simulink model "Problem11"  (R2020a)
settings: Solver=FixedStepDiscrete  StartTime=0.0  StopTime=10.0  FixedStep=1  RelTol=1e-3
settings Model: NumberOfSteps=10  Creator=shweta  LastModifiedBy=shweta

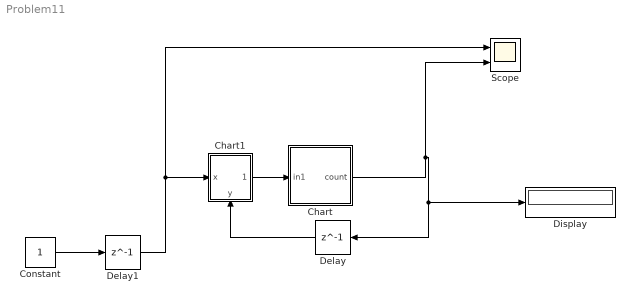
== system Problem11 ==
  Chart : Stateflow chart  TreatAsAtomicUnit=on
  Chart1 : Stateflow chart  TreatAsAtomicUnit=on
      settings: PortSchema="{\"entries\":[{\"content\":{\"sides\":[{\"content\":{\"connectorIds\":[\"In1\"]},\"type\":\"ConnectorPlacement.EquallySpacedRectSide\",\"uuid\":\"73ab95d6-fdc5-46d1-9f3d-9251d1a5c901\"},{\"content\":{\"connectorIds\":[\"Out1\"],\"side\":\"RIGHT\"},\"type\":\"ConnectorPlacement.EquallySpacedRectSide\",\"uuid\":\"b6b0eea8-d45c-469e-b90f-05fc16122799\"},{\"content\":{\"connectorIds\":[],\"side\":\"TOP\"},\"type\":\"ConnectorPlacement.EquallySpacedRectSide\",\"uuid\":\"abd6383a-6df9-4f24-9cd2-85cacf4085cc\"},{\"content\":{\"connectorIds\":[\"In2\"],\"side\":\"BOTTOM\"},\"type\":\"ConnectorPlacement.EquallySpacedRectSide\",\"uuid\":\"4acf616f-2b1a-4d7d-adda-b38e711a4550\"}]},\"type\":\"ConnectorPlacement.EquallySpacedConnector\",\"uuid\":\"c1165d05-06f7-49c3-a608-9e64b2a03931\"}],\"packageUris\":[\"http://schema.mathworks.com/mf0/Connector/19700101\"],\"version\":\"1.0\"}"
  Constant : Constant
  Delay : Delay  DelayLength=1
  Delay1 : Delay  DelayLength=1
  Display : Display
  Scope : Scope  NumInputPorts=2
  wires:
  Chart/1(count) -> Scope/2, Delay/1, Display/1
  Constant/1 -> Delay1/1
  Delay1/1 -> Scope/1, Chart1/1(x)
  Delay/1 -> Chart1/2(y)
  Chart1/1(sum) -> Chart/1(in1)

== stateflow chart Problem11/Chart1 ==
  state adder
    entry:
    sum=x||y;
  (default) -> adder
  data: x input; sum output; y input

== stateflow chart Problem11/Chart ==
  (default) -> (junction 12) : {temp=in1
      | out=0;}
  (junction 19) -> (junction 12)
  (junction 12) -> (junction 14) : {temp=temp+1;
      |
      | out=temp;
      | ;}
  (junction 14) -> (junction 19) [order 1] : [temp<=5]
  (junction 14) -> (junction 18) [order 2] : {count=out;
      | }
  data: count output; temp local; out local; in1 input
